simulink model "simulation"  (R2019b)
settings: Solver=VariableStepAuto  StartTime=0.0  StopTime=5  MaxStep=0.01  RelTol=1e-3
values from neighbouring files (symbols this model uses):
  A = cat(1,cat(2, zeros(2,2),eye(2)), cat(2,-inv(M)*K,-inv(M)*C))    [parameter.m]
  B = cat(1,zeros(2,2),-inv(M)*G)    [parameter.m]
  C0 = cat(2,eye(2),zeros(2,2))    [parameter.m]
  D = zeros(2,2)    [parameter.m]
settings Model: Creator=86189  LastModifiedBy=86189

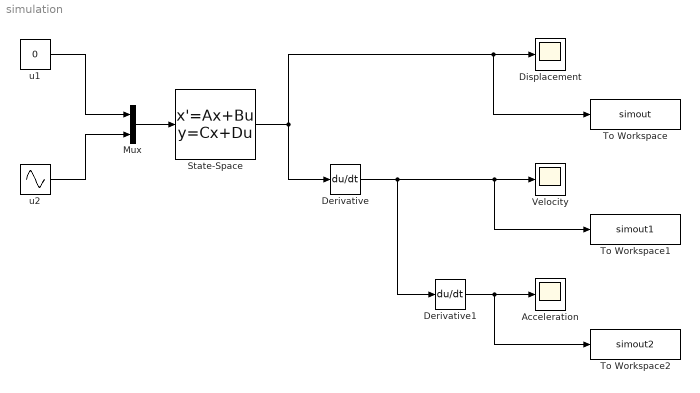
== system simulation ==
  Acceleration : Scope
  Derivative : Derivative
  Derivative1 : Derivative
  Displacement : Scope
  Mux : Mux  Inputs=2
  State-Space : StateSpace  A=A  B=B  C=C0  D=D  InitialCondition=0
  To Workspace : ToWorkspace  VariableName=simout  SaveFormat=Timeseries  SampleTime=-1
  To Workspace1 : ToWorkspace  VariableName=simout1  SaveFormat=Timeseries  SampleTime=-1
  To Workspace2 : ToWorkspace  VariableName=simout2  SaveFormat=Timeseries  SampleTime=-1
  Velocity : Scope
  u1 : Constant  Value=0
  u2 : Sin  Amplitude=2000  Frequency=20  SampleTime=0
  wires:
  State-Space/1 -> To Workspace/1, Displacement/1, Derivative/1
  Derivative/1 -> To Workspace1/1, Velocity/1, Derivative1/1
  Derivative1/1 -> Acceleration/1, To Workspace2/1
  Mux/1 -> State-Space/1
  u1/1 -> Mux/1
  u2/1 -> Mux/2
